simulink model "Q9"  (Simulink 8.5)
settings: Solver=ode45  StartTime=0.0  StopTime=t_paragem  RelTol=1e-3
values from neighbouring files (symbols this model uses):
  dy0 = dy    [e_11.m]    (also in lab2.m)
  y0 = y    [e_11.m]    (also in lab2.m)
undefined symbols (not defined in the file or in its folder): sgn
settings Model: Creator=ricar  LastModifiedBy=Carlos
settings DataIOCC: LimitDataPoints=off  SaveFormat=Dataset  SignalLoggingSaveFormat=Dataset
settings OptimizationCC: ExpressionDepthLimit=128
settings DebuggingCC: UnderspecifiedInitializationDetection=Simplified  MergeDetectMultiDrivingBlocksExec=error  FcnCallInpInsideContextMsg=EnableAllAsError  StateNameClashWarn=none
settings HardwareCC: ProdBitPerPointer=64  ProdLargestAtomicFloat=Float  ProdIntDivRoundTo=Zero  ProdEndianess=LittleEndian  ProdHWDeviceType=Specified
settings ModelReferenceCC: PropagateSignalLabelsOutOfModel=on
settings GRTTargetCC: CombineOutputUpdateFcns=on  GRTInterface=off

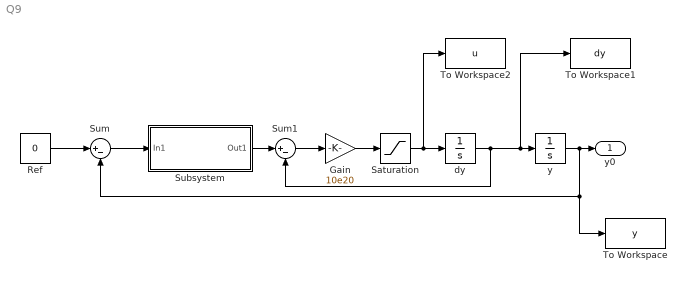
== system Q9 ==
  Gain : Gain  Gain=10e20
  Ref : Constant  Value=0
  Saturation : Saturate  UpperLimit=1  LowerLimit=-1  ZeroCross=off
  Subsystem : Subsystem
  Sum : Sum  Inputs=|+-
  Sum1 : Sum  Inputs=|+-
  To Workspace : ToWorkspace  VariableName=y  SampleTime=-1
  To Workspace1 : ToWorkspace  VariableName=dy  SampleTime=-1
  To Workspace2 : ToWorkspace  VariableName=u  SampleTime=-1
  dy : Integrator  InitialCondition=dy0
  y : Integrator  InitialCondition=y0
  y0 : Outport
  wires:
  Subsystem/1(Out1) -> Sum1/1
  Sum1/1 -> Gain/1
  Gain/1 -> Saturation/1
  y/1 -> To Workspace/1, Sum/2, y0/1
  dy/1 -> To Workspace1/1, y/1, Sum1/2
  Saturation/1 -> To Workspace2/1, dy/1
  Sum/1 -> Subsystem/1(In1)
  Ref/1 -> Sum/1

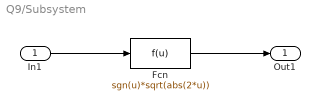
== system Q9/Subsystem ==
  In1 : Inport
  Fcn : Fcn  Expr=sgn(u)*sqrt(abs(2*u))
  Out1 : Outport
  wires:
  In1/1 -> Fcn/1
  Fcn/1 -> Out1/1
